simulink model "Es2_sim"  (R2023a)
settings: Solver=VariableStepAuto  StartTime=0.0  StopTime=10.0  RelTol=1e-3
values from neighbouring files (symbols this model uses):
  x0 = [3;5]    [Es2.m]
settings Model: Creator=Daniil  LastModifiedBy=Daniil

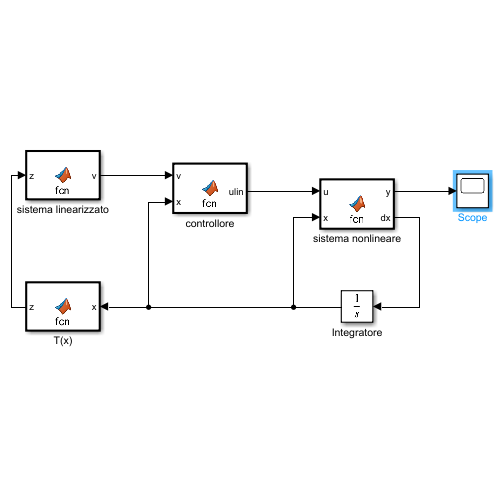
[thumbnail: Simulink's stored preview of the top-level diagram]
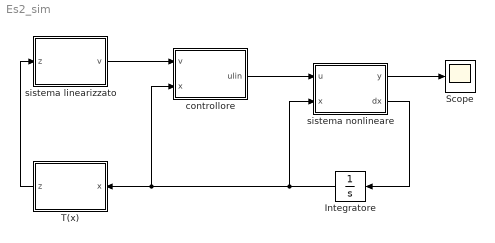
== system Es2_sim ==
  Integratore : Integrator  InitialCondition=x0
  Scope : Scope
  T(x) : MATLAB Function  TreatAsAtomicUnit=on
  controllore : MATLAB Function  TreatAsAtomicUnit=on
  sistema linearizzato : MATLAB Function  TreatAsAtomicUnit=on
  sistema nonlineare : MATLAB Function  TreatAsAtomicUnit=on
  wires:
  sistema nonlineare/2(dx) -> Integratore/1
  Integratore/1 -> sistema nonlineare/2(x), T(x)/1(x), controllore/2(x)
  sistema nonlineare/1(y) -> Scope/1
  controllore/1(ulin) -> sistema nonlineare/1(u)
  sistema linearizzato/1(v) -> controllore/1(v)
  T(x)/1(z) -> sistema linearizzato/1(z)

== matlab function Es2_sim/sistema nonlineare ==
  data: y output; dx output; u input; x input
function [y,dx] = fcn(u,x)
    x1 = x(1);
    x2 = x(2);
    dx = [3*(x1+1)*x1*x2; -4*x2+x1-x2*u+3*u];
y = 2*x1;;

== matlab function Es2_sim/sistema linearizzato ==
  data: z input; v output
function v = fcn(z)
v=[12.5 7.5]*z;

== matlab function Es2_sim/T(x) ==
  data: x input; z output
function z = fcn(x)
    x1=x(1);
    x2=x(2);
    % diffeomorfismo: z=T(x)=[yB; dyB]
    z= [2*x1; 2*x1*x2*(3*x1 + 3)];

== matlab function Es2_sim/controllore ==
  data: v input; ulin output; x input
function ulin = fcn(v,x)
x1=x(1);
x2=x(2);
ulin = (2*x1*(3*x1+3)*(x1-4*x2)-v+x1*x2*(3*x1+3)*(2*x2*(3*x1+3)+6*x1*x2))/(2*x1*(3*x1+3)*(x2-3));
